simulink model "LQG_Regulator"  (R2012b)
settings: Solver=ode45  StartTime=0.0  StopTime=50  RelTol=1e-3
values from neighbouring files (symbols this model uses):
  Initial_conditions = [-1 1 0.5 -0.5 1]    [Problems.m]
  Noise_Gain = 2    [Problems.m]
  RSYS = reg(SYS,K,L)    [Skrypt.m]
  SYS = ss(A, B, C, D)    [Skrypt.m]
settings Model: Creator=Vallen  LastModifiedBy=Vallen

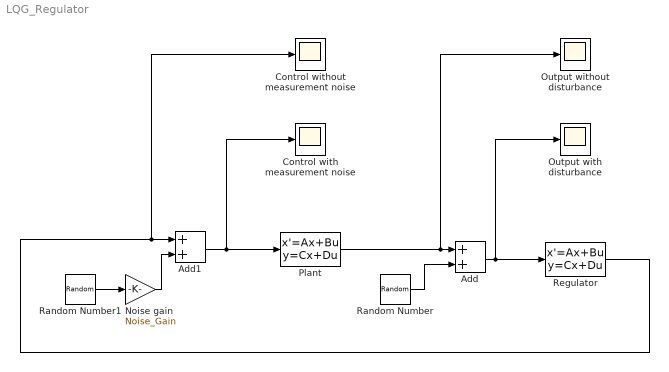
== system LQG_Regulator ==
  Add : Sum
  Add1 : Sum
  Control with measurement noise : Scope
      settings: TimeRange=50
  Control without measurement noise : Scope
      settings: TimeRange=50  SaveName=ScopeData2
  Noise gain : Gain  Gain=Noise_Gain
  Output with disturbance : Scope
      settings: TimeRange=50  SaveName=ScopeData3
  Output without disturbance : Scope
      settings: TimeRange=50
  Plant : StateSpace  A=SYS.A  B=SYS.B  C=SYS.C  D=SYS.D  X0=Initial_conditions
  Random Number : RandomNumber  Variance=0.2  SampleTime=0.1
  Random Number1 : RandomNumber  Variance=0.2  Seed=2  SampleTime=0.1
  Regulator : StateSpace  A=RSYS.A  B=RSYS.B  C=RSYS.C  D=RSYS.D
  wires:
  Plant/1 -> Output without disturbance/1, Add/1
  Random Number/1 -> Add/2
  Random Number1/1 -> Noise gain/1
  Add1/1 -> Control with measurement noise/1, Plant/1
  Add/1 -> Output with disturbance/1, Regulator/1
  Regulator/1 -> Add1/1, Control without measurement noise/1
  Noise gain/1 -> Add1/2
